simulink model "AVC"  (Simulink 7.4)
settings: Solver=ode23tb  StartTime=0.0  StopTime=1  RelTol=1e-3
libraries: powerlib x14, powerlib_extras x1
settings Model: Creator=SIG4  LastModifiedBy=SIG4
settings DataIOCC: SaveOutput=off  SaveTime=off
settings OptimizationCC: InitFltsAndDblsToZero=on  OptimizeModelRefInitCode=on
settings DebuggingCC: SaveWithParameterizedLinksMsg=none  MultiTaskCondExecSysMsg=none  StrictBusMsg=None
settings HardwareCC: ProdIntDivRoundTo=Zero  ProdEndianess=LittleEndian  ProdHWDeviceType=Analog Devices->Blackfin
settings RTWCC: SystemTargetFile=vdsplink_ert.tlc  GenCodeOnly=on  GenerateMakefile=off  TemplateMakefile=vdsplink_ert.tmf  Description=Embedded IDE Link (for use with Analog Devices(TM) VisualDSP++(R)) ERT code generation  ProcessScript=vdsplink_ert_make_rtw_hook  IncludeERTFirstTime=on
settings CodeAppCC: IgnoreCustomStorageClasses=off
settings ERTTgtLinkVDSP: TargetFcnLib=ansi_tfl_table_tmw.mat  TargetFunctionLibrary=ANSI_C  UtilityFuncGeneration=Auto  ERTMultiwordTypeDef=System defined  ERTMultiwordLength=256  MultiwordLength=2048  GenerateFullHeader=on  GenerateSampleERTMain=off  GenerateTestInterfaces=off  IsPILTarget=off  ModelReferenceCompliant=on  ParMdlRefBuildCompliant=off  CompOptLevelCompliant=off  IncludeMdlTerminateFcn=on  GeneratePreprocessorConditionals=Disable all  CombineOutputUpdateFcns=on  SuppressErrorStatus=off  ERTFirstTimeCompliant=off  IncludeFileDelimiter=Auto  ERTCustomFileBanners=on  SupportAbsoluteTime=on  LogVarNameModifier=rt_  MatFileLogging=off  MultiInstanceERTCode=off  SupportNonFinite=on  SupportComplex=on  PurelyIntegerCode=off  SupportContinuousTime=off  SupportNonInlinedSFcns=off  SupportVariableSizeSignals=off  EnableShiftOperators=on  ParenthesesLevel=Nominal  PortableWordSizes=off  ModelStepFunctionPrototypeControlCompliant=on  CPPClassGenCompliant=off  AutosarCompliant=off  GenerateErtSFunction=off  GenerateASAP2=off  ExtMode=off  ExtModeTransport=0  ExtModeStaticAlloc=off  ExtModeStaticAllocSize=1000000  ExtModeTesting=off  ExtModeMexFile=noextcomm  ExtModeIntrfLevel=Level1  InlinedParameterPlacement=NonHierarchical  TargetOS=BareBoardExample  MultiInstanceErrorCode=Error  RateGroupingCode=on  RootIOFormat=Individual arguments  RTWCAPISignals=off  RTWCAPIParams=off  RTWCAPIStates=off  ERTSrcFileBannerTemplate=ert_code_template.cgt  ERTHdrFileBannerTemplate=ert_code_template.cgt  ERTDataSrcFileTemplate=ert_code_template.cgt  ERTDataHdrFileTemplate=ert_code_template.cgt  ERTCustomFileTemplate=example_file_process.tlc  ModuleNamingRule=Unspecified  SignalDisplayLevel=10  ParamTuneLevel=10  GlobalDataDefinition=Auto  DataDefinitionFile=global.c  GlobalDataReference=Auto  DataReferenceFile=global.h  GRTInterface=off  PreserveExpressionOrder=off  PreserveIfCondition=off  ConvertIfToSwitch=off  PreserveExternInFcnDecls=on  EnableUserReplacementTypes=off  MemSecPackage=--- None ---  MemSecDataConstants=Default  MemSecDataIO=Default  MemSecDataInternal=Default  MemSecDataParameters=Default  MemSecFuncInitTerm=Default  MemSecFuncExecute=Default  exportIDEObj=on  ideObjName=VDSP_Obj  oldideObjName=VDSP_Obj  ideObjTimeout=10  oldideObjTimeout=10  ideObjBuildTimeout=1000  oldideObjBuildTimeout=1000  ProfileGenCode=off  profileBy=Tasks  ProfileNumSamples=100  InlineDSPBlks=on  projectOptions=Custom  getCompilerOptions=off  getLinkerOptions=off  systemStackSize=512  buildAction=Build_and_execute  overrunNotificationMethod=None  overrunNotificationFcn=myfunction  oldoverrunNotificationFcn=myfunction  configurePIL=off  configPILBlockAction=Create_PIL_block_build_and_download  DiagnosticActions=warning  debugCompilerOptions=-g  releaseCompilerOptions=-O -Ov100  releaseLinkerOptions=-ip -e
settings SimEventsCC: propDiagAttribOutput=1  propDiagFcnCallOutput=1  propDiagStatOutput=0

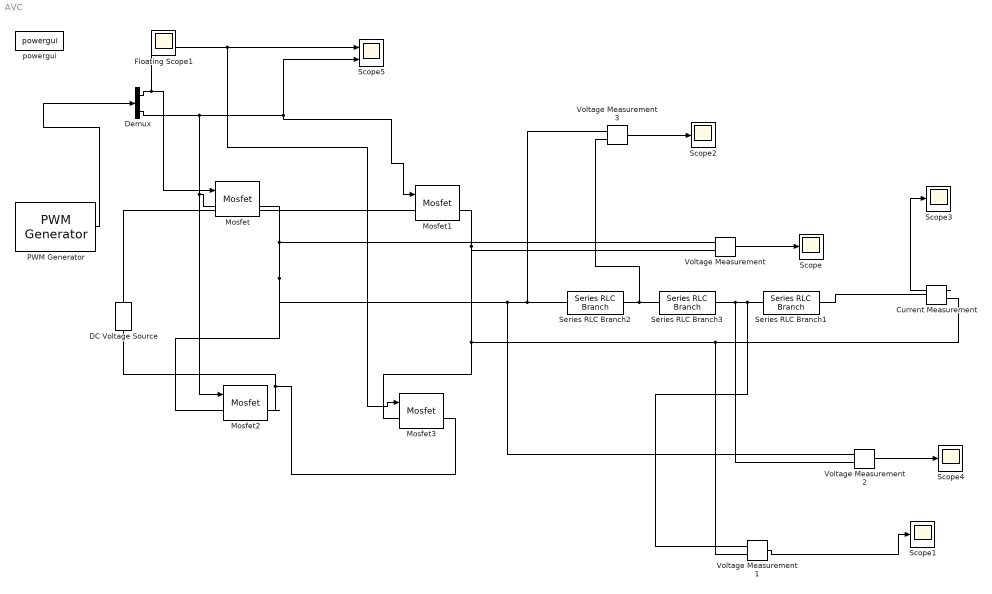
== system AVC ==
  Current Measurement : powerlib/Measurements/Current Measurement  DialogController=POWERSYS.PowerSysDialog  SystemSampleTime=-1  PhasorSimulation=off  OutputType=Complex  PSBequivalent=0
  DC Voltage Source : powerlib/Electrical Sources/DC Voltage Source  DialogController=POWERSYS.PowerSysDialog  SystemSampleTime=-1  Amplitude=150  Measurements=None
  Demux : Demux  Outputs=2
  Mosfet{,1..3} (4 alike) : powerlib/Power Electronics/Mosfet  DialogController=POWERSYS.PowerSysDialog  SystemSampleTime=-1  Ron=.1  Lon=0  Rd=0.01  Vfd=0  IC=0  Rs=1e5  Cs=inf  Measurements=on
  PWM Generator : powerlib_extras/Control  Blocks/PWM Generator  DialogController=POWERSYS.PowerSysDialog  SystemSampleTime=-1  GeneratorMode="1-arm  bridge (2 pulses)"  Fc=10000  Internal=on  mIndex=0.5  Freq=100  Phase=0
  Scope{,1..4} (5 alike) : Scope
      Scope settings: TickLabels=on  TimeRange=0.007680000000000131  YMin=-200  YMax=200
      Scope1 settings: TickLabels=on  YMin=-0.9  YMax=0.9
      Scope2 settings: TickLabels=on  YMin=-200  YMax=200  SaveName=ScopeData3
      Scope3 settings: TickLabels=on  YMin=-0.15  YMax=0.15  SaveName=ScopeData2
      Scope4 settings: TickLabels=on  YMin=-200  YMax=200  SaveName=ScopeData5
  Scope5 : Scope  NumInputPorts=2
      settings: TickLabels=on  YMin=-200~-5  YMax=200~5  SaveName=ScopeData6
  Series RLC Branch1 : powerlib/Elements/Series RLC Branch  DialogController=POWERSYS.PowerSysDialog  PhysicalDomain=powersysdomain  SubClassName=unknown  LeftPortType=p1  RightPortType=p1  LConnTagsString=__new0  RConnTagsString=__new0  BranchType=C  Resistance=1  Inductance=14.2e-3  SetiL0=off  InitialCurrent=0  Capacitance=25e-6  Setx0=off  InitialVoltage=0  Measurements=None
  Series RLC Branch2 : powerlib/Elements/Series RLC Branch  DialogController=POWERSYS.PowerSysDialog  PhysicalDomain=powersysdomain  SubClassName=unknown  LeftPortType=p1  RightPortType=p1  LConnTagsString=__new0  RConnTagsString=__new0  BranchType=L  Resistance=2  Inductance=150e-3  SetiL0=off  InitialCurrent=0  Capacitance=1e-6  Setx0=off  InitialVoltage=0  Measurements=None
  Series RLC Branch3 : powerlib/Elements/Series RLC Branch  DialogController=POWERSYS.PowerSysDialog  PhysicalDomain=powersysdomain  SubClassName=unknown  LeftPortType=p1  RightPortType=p1  LConnTagsString=__new0  RConnTagsString=__new0  BranchType=R  Resistance=50  Inductance=14.2e-3  SetiL0=off  InitialCurrent=0  Capacitance=10e-6  Setx0=off  InitialVoltage=0  Measurements=None
  Voltage Measurement{,1..3} (4 alike) : powerlib/Measurements/Voltage Measurement  DialogController=POWERSYS.PowerSysDialog  SystemSampleTime=-1  PhasorSimulation=off  OutputType=Complex  PSBequivalent=0
  powergui : powerlib/powergui  SystemSampleTime=-1  SimulationMode=Continuous  SampleTime=50e-6  frequency=60  SPID=off  DisableSnubberDevices=off  DisableRonSwitches=off  DisableVfSwitches=off  SwTol=0  Interpol=off  frequencyindice=0  echomessages=off  HookPort=off  DisplayEquations=off  FunctionMessages=off  EnableUseOfTLC=off  x0status=blocks  RestoreLinks=warning  Frange=[0:2:500]  Ylog=off  Xlog=on  ShowGrid=off  save=off  variable=ZData  ZoomFFT=on  StartTime=0.0  cycles=1  DisplayStyle=1  fundamental=60  FreqAxis=off  MaxFrequency=1000  frequencyindicesteady=1  RmsSteady=1  display=off  Ts=0  methode=off
  Floating Scope1 : Scope
      settings: Floating=on  SaveName=ScopeData4
  wires:
  Voltage Measurement3/1 -> Scope2/1
  Voltage Measurement/1 -> Scope/1
  PWM Generator/1 -> Demux/1
  Demux/1 -> Mosfet/1, Scope5/1, Mosfet3/1
  Demux/2 -> Mosfet1/1, Scope5/2, Mosfet2/1
  Voltage Measurement1/1 -> Scope1/1
  Current Measurement/1 -> Scope3/1
  Voltage Measurement2/1 -> Scope4/1
  connections:
  DC Voltage Source/RConn1 -- Mosfet/LConn1 -- Mosfet1/LConn1
  Mosfet1/RConn1 -- Voltage Measurement/LConn2 -- Mosfet3/LConn1 -- Voltage Measurement1/LConn2 -- Current Measurement/RConn1
  Mosfet2/RConn1 -- DC Voltage Source/LConn1 -- Mosfet3/RConn1
  Series RLC Branch2/RConn1 -- Voltage Measurement3/LConn2 -- Series RLC Branch3/LConn1
  Mosfet2/LConn1 -- Voltage Measurement/LConn1 -- Mosfet/RConn1 -- Voltage Measurement2/LConn1 -- Voltage Measurement3/LConn1 -- Series RLC Branch2/LConn1
  Current Measurement/LConn1 -- Series RLC Branch1/RConn1
  Series RLC Branch3/RConn1 -- Voltage Measurement2/LConn2 -- Series RLC Branch1/LConn1 -- Voltage Measurement1/LConn1
